simulink model "lab_2_n_3"  (R2021b)
settings: Solver=VariableStepAuto  StartTime=0.0  StopTime=100.0  RelTol=1e-3
settings Model: Creator=peter  LastModifiedBy=peter

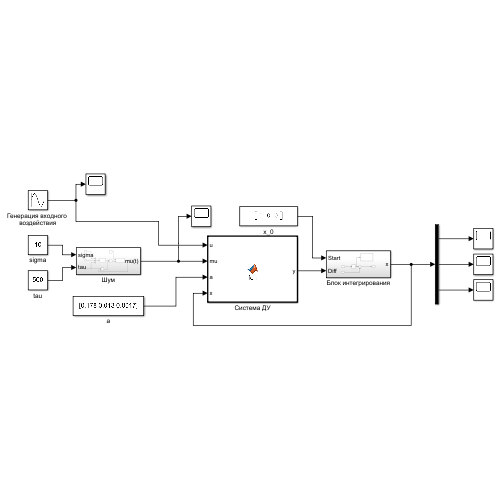
[thumbnail: Simulink's stored preview of the top-level diagram]
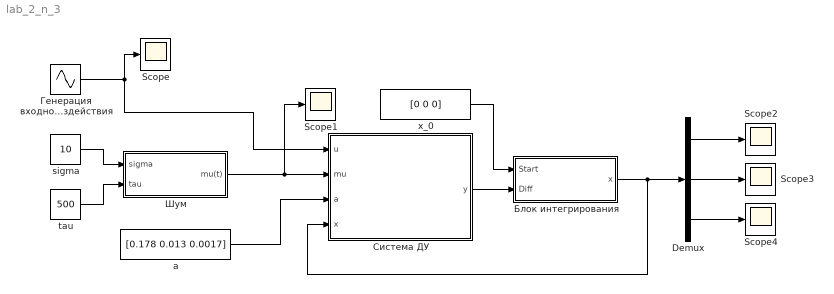
== system lab_2_n_3 ==
  Demux : Demux  Outputs=3
  Scope{,1..4} (5 alike) : Scope
  a : Constant  Value=[0.178 0.013 0.0017]
  sigma : Constant  Value=10
  tau : Constant  Value=500
  x_0 : Constant  Value=[0 0 0]
  Блок интегрирования : Subsystem
  Генерация входного воздействия : Sin  Frequency=0.05  SampleTime=0
  Система ДУ : MATLAB Function  TreatAsAtomicUnit=on
  Шум : Subsystem
  wires:
  Demux/1 -> Scope2/1
  Demux/2 -> Scope3/1
  Demux/3 -> Scope4/1
  Блок интегрирования/1(x) -> Система ДУ/4(x), Demux/1
  x_0/1 -> Блок интегрирования/1(Start)
  Шум/1(mu(t)) -> Система ДУ/2(mu), Scope1/1
  tau/1 -> Шум/2(tau)
  sigma/1 -> Шум/1(sigma)
  Генерация входного воздействия/1 -> Система ДУ/1(u), Scope/1
  a/1 -> Система ДУ/3(a)
  Система ДУ/1(y) -> Блок интегрирования/2(Diff)

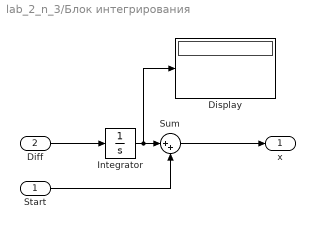
== system lab_2_n_3/Блок интегрирования ==
  Start : Inport
  Diff : Inport  Port=2
  Display : Display
  Integrator : Integrator
  Sum : Sum  Inputs=|++
  x : Outport
  wires:
  Diff/1 -> Integrator/1
  Sum/1 -> x/1
  Integrator/1 -> Display/1, Sum/1
  Start/1 -> Sum/2

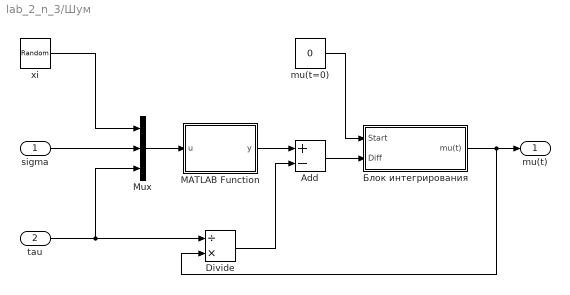
== system lab_2_n_3/Шум ==
  sigma : Inport
  tau : Inport  Port=2
  Add : Sum  Inputs=+-
  Divide : Product  Inputs=/*
  MATLAB Function : MATLAB Function  TreatAsAtomicUnit=on
  Mux : Mux  Inputs=3
  mu(t=0) : Constant  Value=0
  xi : RandomNumber  SampleTime=0.1
  Блок интегрирования : Subsystem
  mu(t) : Outport
  wires:
  mu(t=0)/1 -> Блок интегрирования/1(Start)
  Блок интегрирования/1(mu(t)) -> Divide/2, mu(t)/1
  xi/1 -> Mux/1
  sigma/1 -> Mux/2
  tau/1 -> Mux/3, Divide/1
  Add/1 -> Блок интегрирования/2(Diff)
  Divide/1 -> Add/2
  MATLAB Function/1(y) -> Add/1
  Mux/1 -> MATLAB Function/1(u)

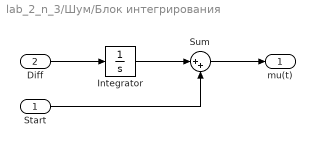
== system lab_2_n_3/Шум/Блок интегрирования ==
  Start : Inport
  Diff : Inport  Port=2
  Integrator : Integrator
  Sum : Sum  Inputs=|++
  mu(t) : Outport
  wires:
  Integrator/1 -> Sum/1
  Sum/1 -> mu(t)/1
  Diff/1 -> Integrator/1
  Start/1 -> Sum/2

== matlab function lab_2_n_3/Система ДУ ==
  data: u input; y output; mu input; a input; x input
function y = fcn(u,mu,a,x)
    dx_1=x(2);
    dx_2=x(3);
    dx_3=u+mu-a(1)*x(1)-a(2)*x(2)-a(3)*x(3);
y = [dx_1, 
    dx_2, 
    dx_3];

== matlab function lab_2_n_3/Шум/MATLAB Function ==
  data: u input; y output
function y = fcn(u)
    xi=u(1);
    sigma=u(2);
    tau=u(3);
    alpha=1/tau;
    k_f=sigma*sqrt(2*alpha);
y = k_f*xi;
